simulink model "green_joint_mit_impedance_model"  (R2023b)
settings: Solver=FixedStepDiscrete  StartTime=0.0  StopTime=0.001  FixedStep=5e-05  RelTol=1e-3
values from neighbouring files (symbols this model uses):
  GJMitPi = 3.1415927410125732    [green_joint_mit_impedance_interface.sldd]
  GJMitTwoPi = 6.2831854820251465    [green_joint_mit_impedance_interface.sldd]
settings Model: DataDictionary=green_joint_mit_impedance_interface.sldd  Creator=user  LastModifiedBy=user
settings OptimizationCC: EnhancedBackFolding=on  PassReuseOutputArgsAs=Individual arguments  OptimizeBlockOrder=speed  DifferentSizesBufferReuse=on  OptimizationCustomize=off  EfficientTunableParamExpr=on
settings DebuggingCC: ParameterPrecisionLossMsg=none  ParameterTunabilityLossMsg=error
settings HardwareCC: ProdBitPerPointer=32  ProdBitPerSizeT=32  ProdBitPerPtrDiffT=32  ProdLargestAtomicInteger=Long  ProdLargestAtomicFloat=Double  ProdWordSize=32  ProdHWDeviceType=ARM Compatible->ARM Cortex  TargetLargestAtomicInteger=Long  TargetLargestAtomicFloat=Double  TargetIntDivRoundTo=Zero  TargetEndianess=LittleEndian  TargetHWDeviceType=ARM Compatible->ARM Cortex  ProdEqTarget=off
settings SFSimCC: MATLABDynamicMemAlloc=off
settings RTWCC: Description=Embedded Coder  SystemTargetFile=ert.tlc  GenCodeOnly=on  TemplateMakefile=ert_default_tmf  GenerateReport=on
settings CodeAppCC: ForceParamTrailComments=on  IgnoreCustomStorageClasses=off  OperatorAnnotations=on  SimulinkDataObjDesc=on  SFDataObjDesc=on  InsertBlockDesc=on
settings ERTTargetCC: TargetLangStandard=C99 (ISO)  CodeInterfacePackaging=Reusable function  ERTCustomFileTemplate=example_file_process.tlc

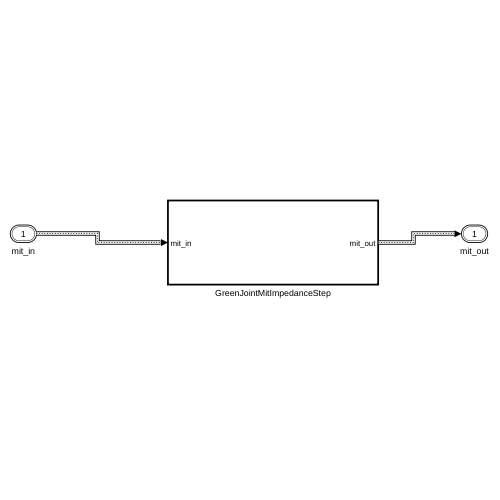
[thumbnail: Simulink's stored preview of the top-level diagram]
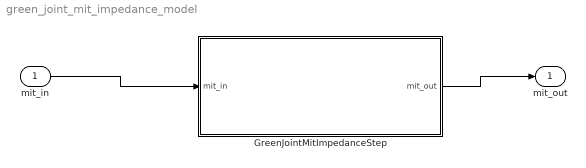
== system green_joint_mit_impedance_model ==
  mit_in : Inport  OutDataTypeStr=Bus: green_joint_mit_input_t  BusOutputAsStruct=on
  GreenJointMitImpedanceStep : Subsystem  TreatAsAtomicUnit=on  RTWFcnName=GreenJointMitImpedanceStep  RTWFileName=GreenJointMitImpedanceStep
      settings: RTWFcnNameOpts=User specified  RTWFileNameOpts=User specified
  mit_out : Outport  OutDataTypeStr=Bus: green_joint_mit_output_t
  wires:
  mit_in/1 -> GreenJointMitImpedanceStep/1(mit_in)
  GreenJointMitImpedanceStep/1(mit_out) -> mit_out/1

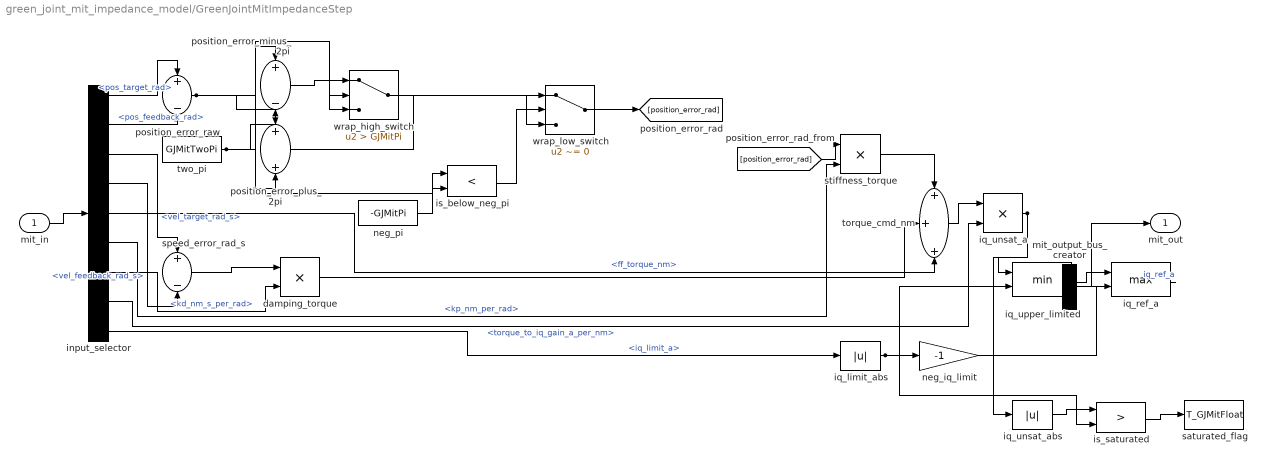
== system green_joint_mit_impedance_model/GreenJointMitImpedanceStep ==
  mit_in : Inport  OutDataTypeStr=Bus: green_joint_mit_input_t  BusOutputAsStruct=on
  damping_torque : Product  OutDataTypeStr=T_GJMitTorque
  input_selector : BusSelector  OutputSignals=pos_target_rad,pos_feedback_rad,vel_target_rad_s,vel_feedback_rad_s,ff_torque_nm,kp_nm_per_rad,kd_nm_s_per_rad,torque_to_iq_gain_a_per_nm,iq_limit_a
  iq_limit_abs : Abs  OutDataTypeStr=T_GJMitCurrent  SaturateOnIntegerOverflow=off
  iq_ref_a : MinMax  Function=max  Inputs=2
  iq_unsat_a : Product  OutDataTypeStr=T_GJMitCurrent
  iq_unsat_abs : Abs  OutDataTypeStr=T_GJMitCurrent  SaturateOnIntegerOverflow=off
  iq_upper_limited : MinMax  Inputs=2
  is_below_neg_pi : RelationalOperator  Operator=<  OutDataTypeStr=boolean  RndMeth=Simplest  InputSameDT=off
  is_saturated : RelationalOperator  Operator=>  OutDataTypeStr=boolean  RndMeth=Simplest  InputSameDT=off
  mit_output_bus_creator : BusCreator  Inputs=1  OutDataTypeStr=Bus: green_joint_mit_output_t  NonVirtualBus=on
  neg_iq_limit : Gain  Gain=-1  ParamDataTypeStr=T_GJMitFloat  OutDataTypeStr=T_GJMitCurrent
  neg_pi : Constant  Value=-GJMitPi  OutDataTypeStr=T_GJMitAngle  SampleTime=-1
  position_error_minus_2pi : Sum  Inputs=+-  OutDataTypeStr=T_GJMitAngle  AccumDataTypeStr=T_GJMitAngle
  position_error_plus_2pi : Sum  OutDataTypeStr=T_GJMitAngle  AccumDataTypeStr=T_GJMitAngle
  position_error_raw : Sum  Inputs=+-  OutDataTypeStr=T_GJMitAngle  AccumDataTypeStr=T_GJMitAngle
  saturated_flag : DataTypeConversion  OutDataTypeStr=T_GJMitFloat  SaturateOnIntegerOverflow=off  RndMeth=Floor
  speed_error_rad_s : Sum  Inputs=+-  OutDataTypeStr=T_GJMitSpeed  AccumDataTypeStr=T_GJMitSpeed
  stiffness_torque : Product  OutDataTypeStr=T_GJMitTorque
  torque_cmd_nm : Sum  Inputs=+++  OutDataTypeStr=T_GJMitTorque  AccumDataTypeStr=T_GJMitTorque
  two_pi : Constant  Value=GJMitTwoPi  OutDataTypeStr=T_GJMitAngle  SampleTime=-1
  wrap_high_switch : Switch  Criteria=u2 > Threshold  Threshold=GJMitPi  OutDataTypeStr=T_GJMitAngle  SaturateOnIntegerOverflow=off  InputSameDT=off
  wrap_low_switch : Switch  Criteria=u2 ~= 0  OutDataTypeStr=T_GJMitAngle  SaturateOnIntegerOverflow=off  InputSameDT=off
  mit_out : Outport  OutDataTypeStr=Bus: green_joint_mit_output_t
  wires:
  mit_in/1 -> input_selector/1
  input_selector/1 -> position_error_raw/1  "<pos_target_rad>"
  input_selector/2 -> position_error_raw/2  "<pos_feedback_rad>"
  position_error_raw/1 -> position_error_minus_2pi/1, position_error_plus_2pi/1, wrap_high_switch/2, wrap_high_switch/3, is_below_neg_pi/1
  two_pi/1 -> position_error_minus_2pi/2, position_error_plus_2pi/2
  position_error_minus_2pi/1 -> wrap_high_switch/1
  neg_pi/1 -> is_below_neg_pi/2
  position_error_plus_2pi/1 -> wrap_low_switch/1
  is_below_neg_pi/1 -> wrap_low_switch/2
  wrap_high_switch/1 -> wrap_low_switch/3
  wrap_low_switch/1 -> [position_error_rad]
  input_selector/3 -> speed_error_rad_s/1  "<vel_target_rad_s>"
  input_selector/4 -> speed_error_rad_s/2  "<vel_feedback_rad_s>"
  [position_error_rad] -> stiffness_torque/1
  input_selector/6 -> stiffness_torque/2  "<kp_nm_per_rad>"
  speed_error_rad_s/1 -> damping_torque/1
  input_selector/7 -> damping_torque/2  "<kd_nm_s_per_rad>"
  stiffness_torque/1 -> torque_cmd_nm/1
  damping_torque/1 -> torque_cmd_nm/2
  input_selector/5 -> torque_cmd_nm/3  "<ff_torque_nm>"
  torque_cmd_nm/1 -> iq_unsat_a/1
  input_selector/8 -> iq_unsat_a/2  "<torque_to_iq_gain_a_per_nm>"
  input_selector/9 -> iq_limit_abs/1  "<iq_limit_a>"
  iq_limit_abs/1 -> neg_iq_limit/1, iq_upper_limited/2, is_saturated/2
  iq_unsat_a/1 -> iq_upper_limited/1, iq_unsat_abs/1
  iq_upper_limited/1 -> iq_ref_a/1
  neg_iq_limit/1 -> iq_ref_a/2
  iq_unsat_abs/1 -> is_saturated/1
  is_saturated/1 -> saturated_flag/1
  iq_ref_a/1 -> mit_output_bus_creator/1  "iq_ref_a"
  mit_output_bus_creator/1 -> mit_out/1
